simulink model "c_lab3sim"  (R2020b)
settings: Solver=FixedStepAuto  StartTime=0.0  StopTime=30  FixedStep=0.001  RelTol=1e-3
settings Model: Creator=musa oğural  LastModifiedBy=musa oğural

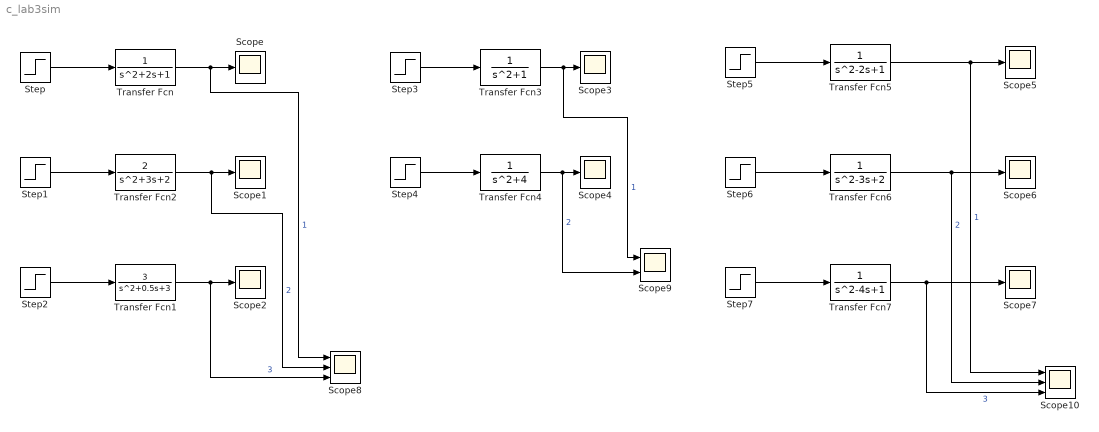
== system c_lab3sim ==
  Scope{,1..7} (8 alike) : Scope
  Scope10 : Scope  NumInputPorts=3
  Scope8 : Scope  NumInputPorts=3
  Scope9 : Scope  NumInputPorts=2
  Step{,1..7} (8 alike) : Step  Time=0  SampleTime=0
  Transfer Fcn : TransferFcn
  Transfer Fcn1 : TransferFcn  Numerator=[3]  Denominator=[1,0.5,3]
  Transfer Fcn2 : TransferFcn  Numerator=[2]  Denominator=[1 3 2]
  Transfer Fcn3 : TransferFcn  Denominator=[1 0 1]
  Transfer Fcn4 : TransferFcn  Denominator=[1 0 4]
  Transfer Fcn5 : TransferFcn  Denominator=[1,-2,1]
  Transfer Fcn6 : TransferFcn  Denominator=[1 -3 2]
  Transfer Fcn7 : TransferFcn  Denominator=[1 -4 1]
  wires:
  Step/1 -> Transfer Fcn/1
  Step3/1 -> Transfer Fcn3/1
  Step4/1 -> Transfer Fcn4/1
  Transfer Fcn4/1 -> Scope9/2, Scope4/1  "2"
  Transfer Fcn7/1 -> Scope10/3, Scope7/1  "3"
  Transfer Fcn6/1 -> Scope10/2, Scope6/1  "2"
  Transfer Fcn5/1 -> Scope10/1, Scope5/1  "1"
  Transfer Fcn/1 -> Scope8/1, Scope/1  "1"
  Step2/1 -> Transfer Fcn1/1
  Transfer Fcn1/1 -> Scope8/3, Scope2/1  "3"
  Step1/1 -> Transfer Fcn2/1
  Transfer Fcn2/1 -> Scope8/2, Scope1/1  "2"
  Transfer Fcn3/1 -> Scope9/1, Scope3/1  "1"
  Step5/1 -> Transfer Fcn5/1
  Step6/1 -> Transfer Fcn6/1
  Step7/1 -> Transfer Fcn7/1
